simulink library "INP_UNSP"  (R2024b)
settings: Solver=VariableStepAuto  StartTime=0.0  StopTime=10.0  RelTol=1e-3
libraries: INP_UNSP_ManOver x1, INP_UNSP_Prep x1
settings Model: Creator=blatak  LastModifiedBy=jmbsp

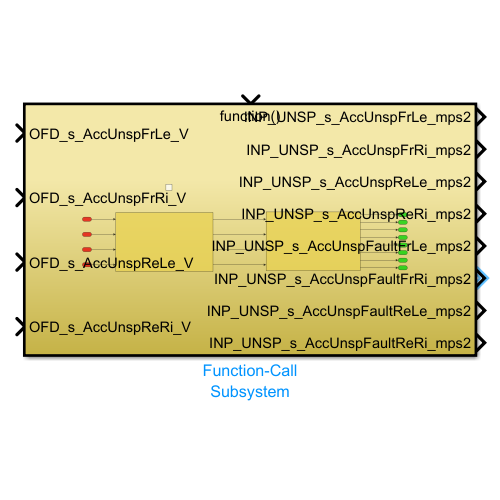
[thumbnail: Simulink's stored preview of the top-level diagram]
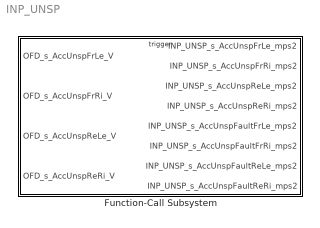
== system INP_UNSP ==
  Function-Call Subsystem : Subsystem  TreatAsAtomicUnit=on

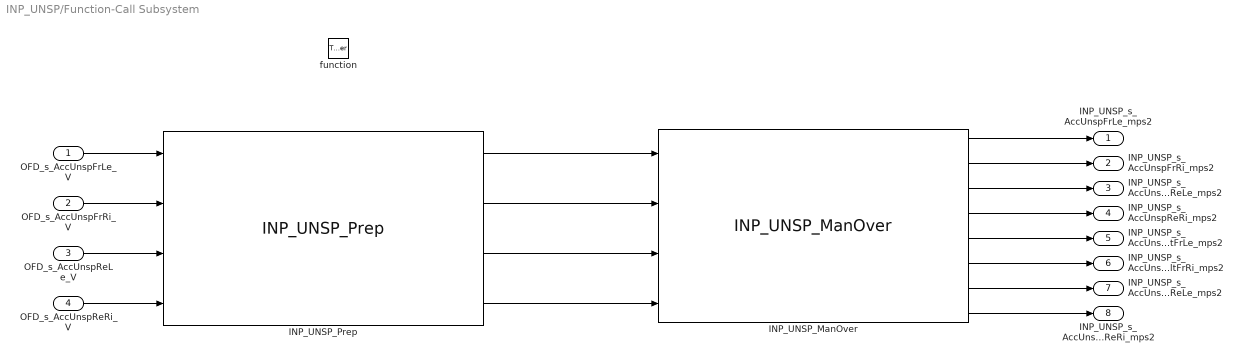
== system INP_UNSP/Function-Call Subsystem ==
  OFD_s_AccUnspFrLe_V : Inport
  OFD_s_AccUnspFrRi_V : Inport  Port=2
  OFD_s_AccUnspReLe_V : Inport  Port=3
  OFD_s_AccUnspReRi_V : Inport  Port=4
  function : TriggerPort  TriggerType=function-call  VariantControl=(inherit)
  INP_UNSP_ManOver : INP_UNSP_ManOver/INP_UNSP_ManOver  SystemSampleTime=-1  VariantActivationTime=update diagram  AllowFlexibleInterface=on  Latency=0  AutoFrameSizeCalculation=off
  INP_UNSP_Prep : INP_UNSP_Prep/INP_UNSP_Prep  SystemSampleTime=-1  VariantActivationTime=update diagram  AllowFlexibleInterface=on  Latency=0  AutoFrameSizeCalculation=off
  INP_UNSP_s_AccUnspFrLe_mps2 : Outport
  INP_UNSP_s_AccUnspFrRi_mps2 : Outport  Port=2
  INP_UNSP_s_AccUnspReLe_mps2 : Outport  Port=3
  INP_UNSP_s_AccUnspReRi_mps2 : Outport  Port=4
  INP_UNSP_s_AccUnspFaultFrLe_mps2 : Outport  Port=5
  INP_UNSP_s_AccUnspFaultFrRi_mps2 : Outport  Port=6
  INP_UNSP_s_AccUnspFaultReLe_mps2 : Outport  Port=7
  INP_UNSP_s_AccUnspFaultReRi_mps2 : Outport  Port=8
  wires:
  INP_UNSP_Prep/1 -> INP_UNSP_ManOver/1
  INP_UNSP_ManOver/8 -> INP_UNSP_s_AccUnspFaultReRi_mps2/1
  INP_UNSP_ManOver/7 -> INP_UNSP_s_AccUnspFaultReLe_mps2/1
  INP_UNSP_ManOver/3 -> INP_UNSP_s_AccUnspReLe_mps2/1
  INP_UNSP_ManOver/2 -> INP_UNSP_s_AccUnspFrRi_mps2/1
  INP_UNSP_ManOver/6 -> INP_UNSP_s_AccUnspFaultFrRi_mps2/1
  INP_UNSP_ManOver/4 -> INP_UNSP_s_AccUnspReRi_mps2/1
  INP_UNSP_ManOver/5 -> INP_UNSP_s_AccUnspFaultFrLe_mps2/1
  INP_UNSP_ManOver/1 -> INP_UNSP_s_AccUnspFrLe_mps2/1
  INP_UNSP_Prep/4 -> INP_UNSP_ManOver/4
  INP_UNSP_Prep/2 -> INP_UNSP_ManOver/2
  OFD_s_AccUnspReRi_V/1 -> INP_UNSP_Prep/4
  OFD_s_AccUnspFrLe_V/1 -> INP_UNSP_Prep/1
  OFD_s_AccUnspReLe_V/1 -> INP_UNSP_Prep/3
  OFD_s_AccUnspFrRi_V/1 -> INP_UNSP_Prep/2
  INP_UNSP_Prep/3 -> INP_UNSP_ManOver/3
